simulink model "Citation_FlightGear_v2"  (R2026a)
settings: Solver=ode5  StopTime=40  FixedStep=0.01  EnableMultiTasking=on
InitFcn:
  | run('initcit.m')
  | run('id_init.m')
values from neighbouring files (symbols this model uses):
  cv1 = 20000    [gear_params.m]
  cv2 = cv1    (= 20000)    [gear_params.m]
  cv3 = 4000    [gear_params.m]
  cv4 = 20000    [gear_params.m]
  deltagmax1 = 0.25    [gear_params.m]
  deltagmax2 = deltagmax1    (= 0.25)    [gear_params.m]
  deltagmax3 = 0.24    [gear_params.m]
  deltagmax4 = 0.02    [gear_params.m]
  kt1 = 525020    [gear_params.m]
  kt2 = kt1    (= 525020)    [gear_params.m]
  kt3 = 457050    [gear_params.m]
  murol = 0.03*10    (= 0.3)    [gear_params.m]
  P1 = 2000    [gear_params.m]
  P2 = P1    (= 2000)    [gear_params.m]
  P3 = 2550    [gear_params.m]
  P4 = 40000    [gear_params.m]
  PL0 = 10000*eye(6)    [id_init.m]
  PM0 = 10000*eye(4)    [id_init.m]
  PN0 = 10000*eye(6)    [id_init.m]
  PX0 = 10000*eye(5)    [id_init.m]
  PY0 = 10000*eye(6)    [id_init.m]
  PZ0 = 10000*eye(4)    [id_init.m]
  thetaL0 = zeros(6,1)    [id_init.m]
  thetaM0 = zeros(4,1)    [id_init.m]
  thetaN0 = zeros(6,1)    [id_init.m]
  thetaX0 = zeros(5,1)    [id_init.m]
  thetaY0 = zeros(6,1)    [id_init.m]
  thetaZ0 = zeros(4,1)    [id_init.m]
  TL = 7.0875e-06    [id_init.m]    (also in plot_comparison_step_4.m = T_var(4))
  TM = 3.2564e-06    [id_init.m]    (also in plot_comparison_step_4.m = T_var(5))
  TN = 5.4692e-07    [id_init.m]    (also in plot_comparison_step_4.m = T_var(6))
  TX = 2.2784e-06    [id_init.m]    (also in plot_comparison_step_4.m = T_var(1))
  TY = 8.0633e-07    [id_init.m]    (also in plot_comparison_step_4.m = T_var(2))
  TZ = 2.8004e-05    [id_init.m]    (also in plot_comparison_step_4.m = T_var(3))
  xl1 = xcg-6.858    [gear_params.m]
  xl2 = xcg-6.858    [gear_params.m]
  xl3 = xcg-2.0752    [gear_params.m]
  xl4 = xcg-12.742    [gear_params.m]
  yl1 = 1.918    [gear_params.m]
  yl2 = -1.918    [gear_params.m]
  yl3 = 0    [gear_params.m]
  yl4 = 0    [gear_params.m]
  zl1 = zcg-1.701    [gear_params.m]
  zl2 = zcg-1.701    [gear_params.m]
  zl3 = zcg-1.7488    [gear_params.m]
  zl4 = zcg-2.78    [gear_params.m]
undefined symbols (not defined in the file or in its folder): chord, Deng, ealphag, ealphas, g0, hDME, hGS, lh, massinit, matbuaf, matdaf, matdam, matdbbf, matdeaf, matdgaf, matdqaf, matduaf, matdwaw, matedhr, mateif, matelhr, matemhr, matemv1, matemv2, matemve, matetam, mateuaf, matfaaf, matfaxl, matff, matibaf, matibb, matibmh, matipaf, matipmh, matiraf, matiuaf, matiwaf, matlaf, matlam, matleaf, matleam, matlgaf, matlqaf, matluaf, matmaaf, matmaam, matmaf, matmam, matmbbf, matmeaf, matmeam, matmgaf, matmqaf, matmrbr, matn1d, matn2d, matnbab, matnbaf, matnbmh ... (+53)
libraries: simulink x12, aerolibfltsims x3, aerolibconvert2 x2, aerolibobsolete x1, aerolibanimutils x1
(part 1 of 5)
settings Model: ExtModeTrigMode=oneshot  ExtModeArmWhenConnect=off  Creator=laurensvaneykeren  LastModifiedBy=eltjo
settings DataIOCC: SignalLoggingSaveFormat=ModelDataLogs  SignalLoggingName=sigsOut
settings OptimizationCC: BooleanDataType=off
settings DebuggingCC: SaveWithParameterizedLinksMsg=none  UnderspecifiedInitializationDetection=Classic  SignalResolutionControl=TryResolveAllWithWarning  MultiTaskDSMMsg=warning  MultiTaskCondExecSysMsg=none
settings HardwareCC: ProdHWDeviceType=32-bit Generic  TargetUnknown=on
settings RTWCC: SystemTargetFile=grt_malloc.tlc  GenCodeOnly=on  TemplateMakefile=grt_malloc_default_tmf
settings GRTTargetCC: UseMalloc=on  CombineOutputUpdateFcns=off  GRTInterface=on

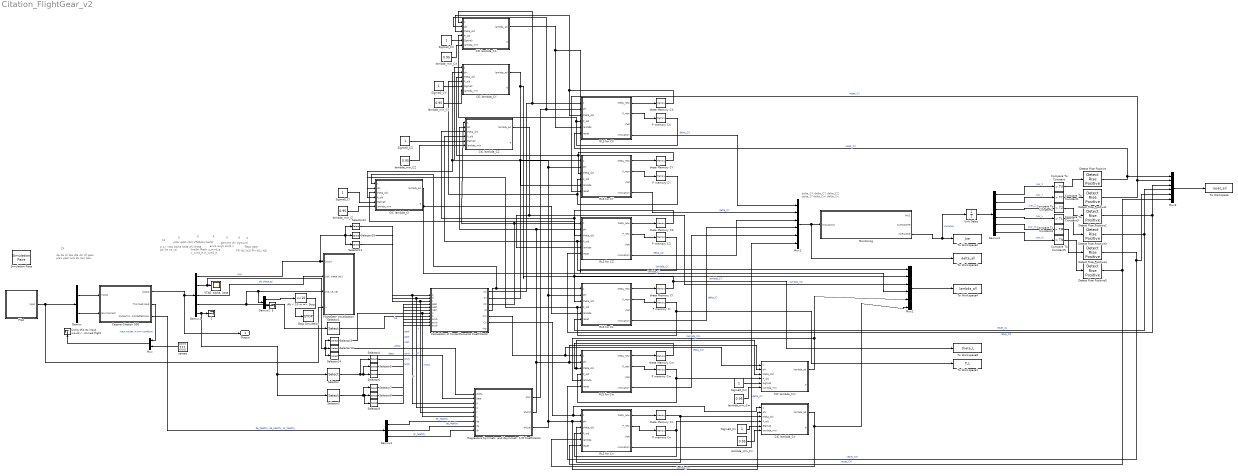
== system Citation_FlightGear_v2 ==
  note: de
      | da
      | dr
      | dte
      | dta
      | dtr
      | df
      | gear
      | pla1
      | pla2
      | turb 8x
      | terr elev
  note: p
      | q
      | r
      | vtas
      | alpha
      | beta
      | phi
      | theta
      | psi
      | he
      | xe
      | ye
  note: pdot
      | qdot
      | rdot
      | VTASdot
      | hedot
  note: hradio
      | Mach
      | u_wind_e
      | v_wind_e
      | w_wind_e
  note: anxb
      | anyb
      | anzb
      | n
  note: gamma
      | chi
      | Vground
  note: flaps
      | gear
  note: FFl
      | N1l
      | N2l
      | FFr
      | N1r
      | N2r
  note: 12
  note: 5
  note: 5
  note: 4
  note: 3
  note: 6
  note: 2
  note: 19
  note: delta_CX
      | delta_CY
      | delta_CZ
      | delta_Cl
      | delta_Cm
      | delta_Cn
  2 : Terminator
  3 : Terminator
  Alt < 10 m => Stop : Fcn  Expr=u<10
  CIC lambda_CX : MATLAB Function  TreatAsAtomicUnit=on
  CIC lambda_CY : MATLAB Function  TreatAsAtomicUnit=on
  CIC lambda_CZ : MATLAB Function  TreatAsAtomicUnit=on
  CIC lambda_Cl : MATLAB Function  TreatAsAtomicUnit=on
  CIC lambda_Cm : MATLAB Function  TreatAsAtomicUnit=on
  CIC lambda_Cn : MATLAB Function  TreatAsAtomicUnit=on
  Calculation of Force/Moments Coefficients : MATLAB Function  TreatAsAtomicUnit=on
  Cessna Citation 500 : Subsystem  mask(Citation Aircraft Model){trimdatafile=}
      mask prompts: trimdatafile "Trim Condition"
      mask init:
      | initcit;
      mask Display:
      | image(imread('Citation.jpg'))
      | port_label('input', 1, 'Inputs')
      | port_label('input', 2, 'Environment')
      | port_label('output', 1, 'Outputs')
      | port_label('output', 2, 'Trim inputs')
  Compare To Constant : simulink/Logic and Bit Operations/Compare To Constant  relop=>  const=TX  OutDataTypeStr=boolean
  Compare To Constant1 : simulink/Logic and Bit Operations/Compare To Constant  relop=>  const=TY  OutDataTypeStr=boolean
  Compare To Constant2 : simulink/Logic and Bit Operations/Compare To Constant  relop=>  const=TZ  OutDataTypeStr=boolean
  Compare To Constant3 : simulink/Logic and Bit Operations/Compare To Constant  relop=>  const=TL  OutDataTypeStr=boolean
  Compare To Constant4 : simulink/Logic and Bit Operations/Compare To Constant  relop=>  const=TM  OutDataTypeStr=boolean
  Compare To Constant5 : simulink/Logic and Bit Operations/Compare To Constant  relop=>  const=TN  OutDataTypeStr=boolean
  Demux : Demux  Outputs=[10 9]
      settings: DisplayOption=none
  Demux1 : Demux  Outputs=[3 3 3 3 25]
      settings: DisplayOption=none
  Demux2 : Demux  Outputs=[1 2]
  Demux3 : Demux  Outputs=3
  Demux4 : Demux  Outputs=6
  Detect Rise Positive{,1..5} (6 alike) : simulink/Logic and Bit Operations/Detect Rise Positive  vinit=0  OutDataTypeStr=boolean
  FlightGear Visualisation : Subsystem
  Monitoring : Subsystem
  Mux : Mux  Inputs=2
  Mux1 : Mux  Inputs=6
  Mux2 : Mux  Inputs=6
  Mux3 : Mux  Inputs=6
  P memory CX : Memory  InitialCondition=PX0
  P memory CY : Memory  InitialCondition=PY0
  P memory CZ : Memory  InitialCondition=PZ0
  P memory Cl : Memory  InitialCondition=PL0
  P memory Cm : Memory  InitialCondition=PM0
  P memory Cn : Memory  InitialCondition=PN0
  Pilot : Subsystem
  RLS for CL : MATLAB Function  TreatAsAtomicUnit=on
  RLS for CX : MATLAB Function  TreatAsAtomicUnit=on
  RLS for CY : MATLAB Function  TreatAsAtomicUnit=on
  RLS for CZ : MATLAB Function  TreatAsAtomicUnit=on
  RLS for Cm : MATLAB Function  TreatAsAtomicUnit=on
  RLS for Cn : MATLAB Function  TreatAsAtomicUnit=on
  Regressors Symmetr. and Asymmetr. F/M Coefficients : MATLAB Function  TreatAsAtomicUnit=on
  Selector : Selector  InputPortWidth=25  IndexOptions=Index vector (dialog)  Indices=[1 2 3]  OutputSizes=1
  Selector1 : Selector  InputPortWidth=3  IndexOptions=Index vector (dialog)  Indices=1  OutputSizes=1
  Selector{5,8,10,13} (4 alike) : Selector  InputPortWidth=3  IndexOptions=Index vector (dialog)  Indices=[2]  OutputSizes=1
  Selector{6,9,11,14} (4 alike) : Selector  InputPortWidth=3  IndexOptions=Index vector (dialog)  Indices=[3]  OutputSizes=1
  Selector{3..4,7,12} (4 alike) : Selector  InputPortWidth=3  IndexOptions=Index vector (dialog)  Indices=[1]  OutputSizes=1
  Selector2 : Selector  InputPortWidth=25  IndexOptions=Index vector (dialog)  Indices=[11 12 13]  OutputSizes=1
  Sigma0_CX : Constant
  Sigma0_CY : Constant
  Sigma0_CZ : Constant
  Sigma0_Cl : Constant
  Sigma0_Cm : Constant
  Sigma0_Cn : Constant
  Simulation Pace : aerolibanimutils/Simulation Pace  SimulationPace=1  SleepMode=MATLAB Thread  OutputPaceError=off  SampleTime=-1
      settings: AttributesFormatString=%<SimulationPace> sec/sec
  Stop Simulation : Stop
  To Workspace : ToWorkspace  VariableName=reset_all  SaveFormat=Timeseries  SampleTime=-1
  To Workspace1 : ToWorkspace  VariableName=P_L  SaveFormat=Timeseries  SampleTime=-1
  To Workspace2 : ToWorkspace  VariableName=Jvar  SaveFormat=Timeseries  SampleTime=-1
  To Workspace3 : ToWorkspace  VariableName=delta_all  SaveFormat=Timeseries  SampleTime=-1
  To Workspace4 : ToWorkspace  VariableName=lambda_all  SaveFormat=Timeseries  SampleTime=-1
  To Workspace8 : ToWorkspace  VariableName=theta_L  SaveFormat=Timeseries  SampleTime=-1
  Unit Delay : UnitDelay  SampleTime=0.01
  Using this as input would result in trimmed flight : Terminator
  "VTAS, alpha, beta" : Scope
      settings: ActiveDisplayYMinimum=-192.0765592563377  ActiveDisplayYMaximum=190.51852643229006  DataLoggingVariableName=ScopeData7
  lambda_min_CX : Constant  Value=0.95
  lambda_min_CY : Constant  Value=0.95
  lambda_min_CZ : Constant  Value=0.95
  lambda_min_Cl : Constant  Value=0.95
  lambda_min_Cm : Constant  Value=0.95
  lambda_min_Cn : Constant  Value=0.95
  theta Memory CX : Memory  InitialCondition=thetaX0
  theta Memory CY : Memory  InitialCondition=thetaY0
  theta Memory CZ : Memory  InitialCondition=thetaZ0
  theta Memory Cl : Memory  InitialCondition=thetaL0
  theta Memory Cm : Memory  InitialCondition=thetaM0
  theta Memory Cn : Memory  InitialCondition=thetaN0
  zeroes : Constant  Value=[0 0 0 0 0 0 0 0 0]
  Output : Outport
  wires:
  Demux/1 -> Cessna Citation 500/1(Inputs)
  Cessna Citation 500/1(output) -> Demux1/1, Output/1
  Demux/2 -> Cessna Citation 500/2(Environment)
  Cessna Citation 500/2(Trimmed input) -> Mux/1  "Input values in trim condition"
  zeroes/1 -> Mux/2
  Mux/1 -> Using this as input would result in trimmed flight/1
  Demux1/1 -> Selector11/1, Selector12/1, Selector10/1, FlightGear Visualisation/1("[p,q,r]")  "p,q,r"
  Demux1/2 -> Selector14/1, Selector3/1, Selector13/1, "VTAS, alpha, beta"/1
  Alt < 10 m => Stop/1 -> Stop Simulation/1
  Demux1/5 -> Selector2/1, Selector/1, 2/1
  Demux1/4 -> Selector1/1, Demux2/1, FlightGear Visualisation/3("[he, xe, ye]")
  Demux2/1 -> Alt < 10 m => Stop/1
  Pilot/1(Input) -> FlightGear Visualisation/4(u), Demux/1
  Demux2/2 -> 3/1
  Demux1/3 -> FlightGear Visualisation/2(" [phi, theta, psi]")  "phi,theta,psi"
  Cessna Citation 500/3(Outport SysID Deflections) -> Demux3/1  "de_healthy, da_healthy, dr_healthy"
  Selector1/1 -> Calculation of Force/Moments Coefficients/8(h)  "he"
  Selector3/1 -> Regressors Symmetr. and Asymmetr. F/M Coefficients/6(V), Calculation of Force/Moments Coefficients/7(V)  "VTAS"
  Selector/1 -> Selector4/1, Selector5/1, Selector6/1
  Selector4/1 -> Calculation of Force/Moments Coefficients/4(pdot)  "pdot"
  Selector5/1 -> Calculation of Force/Moments Coefficients/5(qdot)  "qdot"
  Selector6/1 -> Calculation of Force/Moments Coefficients/6(rdot)  "rdot"
  Selector7/1 -> Calculation of Force/Moments Coefficients/9(anxb)  "anxb"
  Selector9/1 -> Calculation of Force/Moments Coefficients/11(anzb)  "anzb"
  Selector8/1 -> Calculation of Force/Moments Coefficients/10(anyb)  "anyb"
  Selector2/1 -> Selector9/1, Selector8/1, Selector7/1
  Selector12/1 -> Regressors Symmetr. and Asymmetr. F/M Coefficients/3(p), Calculation of Force/Moments Coefficients/1(p)  "p"
  Selector10/1 -> Regressors Symmetr. and Asymmetr. F/M Coefficients/4(q), Calculation of Force/Moments Coefficients/2(q)  "q"
  Selector11/1 -> Regressors Symmetr. and Asymmetr. F/M Coefficients/5(r), Calculation of Force/Moments Coefficients/3(r)  "r"
  Selector13/1 -> Regressors Symmetr. and Asymmetr. F/M Coefficients/1(alpha)  "alpha"
  Selector14/1 -> Regressors Symmetr. and Asymmetr. F/M Coefficients/2(beta)  "beta"
  Demux3/1 -> Regressors Symmetr. and Asymmetr. F/M Coefficients/7(de)  "de_healthy"
  Demux3/2 -> Regressors Symmetr. and Asymmetr. F/M Coefficients/8(da)  "da_healthy"
  Demux3/3 -> Regressors Symmetr. and Asymmetr. F/M Coefficients/9(dr)  "dr_healthy"
  Regressors Symmetr. and Asymmetr. F/M Coefficients/3(phiLat) -> CIC lambda_Cn/2(phi), RLS for Cn/2(phi), RLS for CL/2(phi), RLS for CY/2(phi), CIC lambda_Cl/2(phi), CIC lambda_CY/2(phi)
  RLS for Cn/1(theta_new) -> theta Memory Cn/1
  theta Memory Cn/1 -> RLS for Cn/3(theta_old), CIC lambda_Cn/3(theta_old)
  RLS for Cn/2(P_new) -> P memory Cn/1
  P memory Cn/1 -> RLS for Cn/4(P_old), CIC lambda_Cn/4(P_old)
  Calculation of Force/Moments Coefficients/1(CX) -> CIC lambda_CX/1(z), RLS for CX/1(z)
  P memory CX/1 -> CIC lambda_CX/4(P_old), RLS for CX/4(P_old)
  theta Memory CX/1 -> CIC lambda_CX/3(theta_old), RLS for CX/3(theta_old)
  RLS for CX/2(P_new) -> P memory CX/1
  RLS for CX/1(theta_new) -> theta Memory CX/1
  Regressors Symmetr. and Asymmetr. F/M Coefficients/1(phiX) -> CIC lambda_CX/2(phi), RLS for CX/2(phi)
  P memory CY/1 -> CIC lambda_CY/4(P_old), RLS for CY/4(P_old)
  theta Memory CY/1 -> CIC lambda_CY/3(theta_old), RLS for CY/3(theta_old)
  RLS for CY/2(P_new) -> P memory CY/1
  RLS for CY/1(theta_new) -> theta Memory CY/1
  Calculation of Force/Moments Coefficients/2(CY) -> RLS for CY/1(z), CIC lambda_CY/1(z)
  P memory CZ/1 -> RLS for CZ/4(P_old), CIC lambda_CZ/4(P_old)
  theta Memory CZ/1 -> CIC lambda_CZ/3(theta_old), RLS for CZ/3(theta_old)
  CIC lambda_CZ/1(lambda_ad) -> RLS for CZ/5(lambda), Mux2/3  "lambda_CZ"
  RLS for CZ/2(P_new) -> P memory CZ/1
  RLS for CZ/1(theta_new) -> theta Memory CZ/1
  Calculation of Force/Moments Coefficients/3(CZ) -> RLS for CZ/1(z), CIC lambda_CZ/1(z)
  Regressors Symmetr. and Asymmetr. F/M Coefficients/2(phiZM) -> CIC lambda_Cm/2(phi), RLS for Cm/2(phi), RLS for CZ/2(phi), CIC lambda_CZ/2(phi)
  P memory Cl/1 -> To Workspace1/1, CIC lambda_Cl/4(P_old), RLS for CL/4(P_old)
  theta Memory Cl/1 -> To Workspace8/1, RLS for CL/3(theta_old), CIC lambda_Cl/3(theta_old)
  CIC lambda_Cl/1(lambda_ad) -> Mux2/4, RLS for CL/5(lambda)  "lambda_Cl"
  RLS for CL/2(P_new) -> P memory Cl/1
  RLS for CL/1(theta_new) -> theta Memory Cl/1
  P memory Cm/1 -> RLS for Cm/4(P_old), CIC lambda_Cm/4(P_old)
  theta Memory Cm/1 -> CIC lambda_Cm/3(theta_old), RLS for Cm/3(theta_old)
  RLS for Cm/2(P_new) -> P memory Cm/1
  RLS for Cm/1(theta_new) -> theta Memory Cm/1
  Calculation of Force/Moments Coefficients/4(Cl) -> CIC lambda_Cl/1(z), RLS for CL/1(z)
  Calculation of Force/Moments Coefficients/5(Cm) -> CIC lambda_Cm/1(z), RLS for Cm/1(z)
  Calculation of Force/Moments Coefficients/6(Cn) -> CIC lambda_Cn/1(z), RLS for Cn/1(z)
  RLS for CX/4(innovation) -> Mux1/1  "delta_CX"
  RLS for CY/4(innovation) -> Mux1/2  "delta_CY"
  RLS for CZ/4(innovation) -> Mux1/3  "delta_CZ"
  RLS for CL/4(innovation) -> Mux1/4  "delta_Cl"
  RLS for Cm/4(innovation) -> Mux1/5  "delta_Cm"
  RLS for Cn/4(innovation) -> Mux1/6  "delta_Cn"
  Mux1/1 -> To Workspace3/1, Monitoring/1(innovations)
  Sigma0_CX/1 -> CIC lambda_CX/5(Sigma0)
  lambda_min_CX/1 -> CIC lambda_CX/6(lambda_min)
  CIC lambda_CX/1(lambda_ad) -> Mux2/1, RLS for CX/5(lambda)  "lambda_CX"
  Sigma0_CY/1 -> CIC lambda_CY/5(Sigma0)
  lambda_min_CY/1 -> CIC lambda_CY/6(lambda_min)
  CIC lambda_CY/1(lambda_ad) -> Mux2/2, RLS for CY/5(lambda)  "lambda_CY"
  Sigma0_CZ/1 -> CIC lambda_CZ/5(Sigma0)
  lambda_min_CZ/1 -> CIC lambda_CZ/6(lambda_min)
  Sigma0_Cl/1 -> CIC lambda_Cl/5(Sigma0)
  lambda_min_Cl/1 -> CIC lambda_Cl/6(lambda_min)
  Sigma0_Cm/1 -> CIC lambda_Cm/5(Sigma0)
  lambda_min_Cm/1 -> CIC lambda_Cm/6(lambda_min)
  CIC lambda_Cm/1(lambda_ad) -> Mux2/5, RLS for Cm/5(lambda)  "lambda_Cm"
  Sigma0_Cn/1 -> CIC lambda_Cn/5(Sigma0)
  lambda_min_Cn/1 -> CIC lambda_Cn/6(lambda_min)
  CIC lambda_Cn/1(lambda_ad) -> Mux2/6, RLS for Cn/5(lambda)  "lambda_Cn"
  Monitoring/3(VARIANCE) -> Unit Delay/1, To Workspace2/1  "Variance"
  Mux2/1 -> To Workspace4/1
  Demux4/1 -> Compare To Constant/1  "Jvar_X"
  Demux4/2 -> Compare To Constant1/1  "Jvar_Y"
  Demux4/3 -> Compare To Constant2/1  "Jvar_Z"
  Demux4/4 -> Compare To Constant3/1  "Jvar_L"
  Demux4/5 -> Compare To Constant4/1  "Jvar_M"
  Demux4/6 -> Compare To Constant5/1  "Jvar_N"
  Compare To Constant/1 -> Detect Rise Positive/1
  Compare To Constant1/1 -> Detect Rise Positive1/1
  Compare To Constant2/1 -> Detect Rise Positive2/1
  Compare To Constant3/1 -> Detect Rise Positive3/1
  Compare To Constant5/1 -> Detect Rise Positive5/1
  Compare To Constant4/1 -> Detect Rise Positive4/1
  Detect Rise Positive/1 -> RLS for CX/6(reset), Mux3/1  "reset_CX"
  Detect Rise Positive1/1 -> Mux3/2, RLS for CY/6(reset)  "reset_CY"
  Detect Rise Positive2/1 -> RLS for CZ/6(reset), Mux3/3  "reset_CZ"
  Detect Rise Positive3/1 -> RLS for CL/6(reset), Mux3/4  "reset_CL"
  Detect Rise Positive4/1 -> Mux3/5, RLS for Cm/6(reset)  "reset_CM"
  Detect Rise Positive5/1 -> RLS for Cn/6(reset), Mux3/6  "reset_CN"
  Mux3/1 -> To Workspace/1
  Unit Delay/1 -> Demux4/1

== system Citation_FlightGear_v2/Cessna Citation 500 ==
  note: p
      | q
      | r
      | vtas
      | alpha
      | beta
      | phi
      | theta
      | psi
      | he
      | xe
      | ye
  note: de
      | da
      | dr
      | dte
      | dta
      | dtr
      | df
      | gear
      | pla1
      | pla2
  note: pdot
      | qdot
      | rdot
      | VTASdot
      | hedot
  note: hradio
      | Mach
      | u_wind_e
      | v_wind_e
      | w_wind_e
  note: anxb
      | anyb
      | anzb
      | n
  note: gamma
      | chi
      | Vground
  note: turb 8x
      | terr_elev
  note: flaps
      | gear
  note: de
      | da
      | dr
      | dte
      | dta
      | dtr
      | df
      | gear
      | pla1
      | pla2
  note: FFl
      | N1l
      | N2l
      | FFr
      | N1r
      | N2r
  Inputs : Inport
  Environment : Inport  Port=2
  Actuators : Subsystem
  Citation model DASMAT : Subsystem
  Controllers : Subsystem
  Demux4 : Demux  Outputs=[8 2]
      settings: DisplayOption=none
  Mux1 : Mux  Inputs=7
  Mux2 : Mux  Inputs=2
  trim conditions : Subsystem
  ua sel : Selector  IndexOptions=Index vector (dialog)  Indices=[5 6]  OutputSizes=1
  xdot sel : Selector  IndexOptions=Index vector (dialog)  Indices=[1 2 3 4 10]  OutputSizes=1
  yacc sel : Selector  IndexOptions=Index vector (dialog)  Indices=[4 5 6 15]  OutputSizes=1
  yair sel : Selector  IndexOptions=Index vector (dialog)  Indices=[6 9 22 23 24]  OutputSizes=1
  yfp sel : Selector  IndexOptions=Index vector (dialog)  Indices=[1 2 15]  OutputSizes=1
  ypp sel : Selector  IndexOptions=Index vector (dialog)  Indices=[2 3 4 13 14 15]  OutputSizes=1
  output : Outport
  Trimmed input : Outport  Port=2
  Outport SysID Deflections : Outport  Port=3
  wires:
  Mux1/1 -> output/1
  Citation model DASMAT/1(x) -> Mux1/1, Controllers/1(state)
  Inputs/1 -> Controllers/2(inputs)
  Demux4/1 -> Citation model DASMAT/1(ua), ua sel/1
  Demux4/2 -> Citation model DASMAT/2(ut)
  Environment/1 -> Citation model DASMAT/3(Environment)
  Citation model DASMAT/3(yair) -> yair sel/1
  yair sel/1 -> Mux1/3
  Citation model DASMAT/2(xdot) -> xdot sel/1
  xdot sel/1 -> Mux1/2
  yacc sel/1 -> Mux1/4
  Citation model DASMAT/4(yacc) -> yacc sel/1
  yfp sel/1 -> Mux1/5
  Citation model DASMAT/5(yfp) -> yfp sel/1
  Actuators/1(Out) -> Demux4/1
  trim conditions/1(ua) -> Mux2/1
  trim conditions/2(ut) -> Mux2/2
  Mux2/1 -> Trimmed input/1
  Controllers/1(control inputs) -> Actuators/1(In)
  ua sel/1 -> Mux1/7
  Citation model DASMAT/6(ypp) -> ypp sel/1
  ypp sel/1 -> Mux1/6
  Actuators/2(Outport SysID Deflections) -> Outport SysID Deflections/1

== system Citation_FlightGear_v2/FlightGear Visualisation ==
  "[p,q,r]" : Inport
  " [phi, theta, psi]" : Inport  Port=2
  "[he, xe, ye]" : Inport  Port=3
  u : Inport  Port=4
  Constant : Constant  Value=0
  Generate Run Script : aerolibfltsims/Generate Run Script  Architecture=Win64  dataFlow=Send  GeometryModelName=Yak-36  AirportId=KSFO  RunwayId=10L  InitialAltitude=7224  InitialHeading=113  OffsetDistance=4.72  OffsetAzimuth=0  InstallScenery=off  DisableShaders=off  OriginAddress=127.0.0.1  DestinationPort=5502  OriginPort=5505  LocalAddress=127.0.0.1  OutputFileName=runfg30.bat  FlightGearBaseDirectory=D:\Program Files\FlightGear3.0
  "P, Q, R" : Scope
      settings: ActiveDisplayYMinimum=-2.789820175659862  ActiveDisplayYMaximum=3.3807681055005783  DataLoggingVariableName=ScopeData2
  Send net_fdm Packet to FlightGear : aerolibfltsims/Send net_fdm Packet to FlightGear  DestinationIpAddress=127.0.0.1  DestinationPort=5502  LocalIpPort=-1  varLen=off  SampleTime=-1
  Subsystem : Subsystem
  Sum1 : Sum  Inputs=|++
  "h, posN,posE " : Scope
      settings: TimeSpan=10  ActiveDisplayYMinimum=-20000  ActiveDisplayYMaximum=10000  DataLoggingVariableName=ScopeData5
  "h, posN,posE, offsets" : Constant  Value=[0 -1000 2000]
  phi,theta,psi : Scope
      settings: ActiveDisplayYMinimum=-14.69567  ActiveDisplayYMaximum=1.72975  DataLoggingVariableName=ScopeData3
  wires:
  "h, posN,posE, offsets"/1 -> Sum1/2
  Sum1/1 -> "h, posN,posE "/1, Subsystem/3(Xe)
  Constant/1 -> Subsystem/4(href)
  u/1 -> Subsystem/5(u)
  Subsystem/1(FG Packet) -> Send net_fdm Packet to FlightGear/1
  "[he, xe, ye]"/1 -> Sum1/1
  "[p,q,r]"/1 -> "P, Q, R"/1, Subsystem/1(pqr)
  " [phi, theta, psi]"/1 -> phi,theta,psi/1, Subsystem/2(phi theta psi)

== system Citation_FlightGear_v2/Monitoring ==
  note: MA2 = moving average of the squared innovation
      | AUTOCORR = autocorrelation function
      | VARIANCE = spectral analysis
  innovations : Inport
  Monitoring Metrics : MATLAB Function  TreatAsAtomicUnit=on
  Zero-Order Hold : ZeroOrderHold  SampleTime=0.01
  MA2 : Outport
  AUTOCORR : Outport  Port=2
  VARIANCE : Outport  Port=3
  wires:
  innovations/1 -> Zero-Order Hold/1
  Zero-Order Hold/1 -> Monitoring Metrics/1(innovations)
  Monitoring Metrics/1(MA2) -> MA2/1
  Monitoring Metrics/2(AUTOCORR) -> AUTOCORR/1
  Monitoring Metrics/3(VARIANCE) -> VARIANCE/1

== system Citation_FlightGear_v2/Pilot ==
  note: de
      | da
      | dr
      | dte
      | dta
      | dtr
      | df
      | gear
      | pla1
      | pla2
      | turb 8x
      | terr elev
  Virtual Joystick (if you don't have a real one!) : Subsystem
  Input : Outport
  wires:
  Virtual Joystick (if you don't have a real one!)/1(Virtual joystick input) -> Input/1

== system Citation_FlightGear_v2/Cessna Citation 500/Actuators ==
  note: de
      | da
      | dr
      | dte
      | dta
      | dtr
      | df
      | gear
      | pla1
      | pla2
  note: de
      | da
      | dr
      | dte
      | dta
      | dtr
      | df
      | gear
      | pla1
      | pla2
  In : Inport
  Add : Sum
  Constant : Constant  Value=-0.28
  Demux : Demux  Outputs=10
      settings: DisplayOption=none
  Failure Activation : Step  Time=100  SampleTime=0
  Gain : Gain  Gain=0.5
  Mux : Mux  Inputs=10
  Mux1 : Mux  Inputs=3
  Switch : Switch  Criteria=u2 > Threshold  Threshold=0.5  SaturateOnIntegerOverflow=off  InputSameDT=off
  To Workspace : ToWorkspace  VariableName=failure_activation  SaveFormat=Timeseries  SampleTime=-1
      settings: Save2DSignal=2-D array (concatenate along first dimension)
  da : Subsystem
  da limits : Saturate  UpperLimit=0.65  LowerLimit=-0.65
  de : Subsystem
  de limits : Saturate  UpperLimit=0.26  LowerLimit=-0.35
  dr : Subsystem
  dr limits : Saturate  UpperLimit=0.38  LowerLimit=-0.38
  flaps : Subsystem
  gear : Subsystem
  Out : Outport
  Outport SysID Deflections : Outport  Port=2
  wires:
  In/1 -> Demux/1
  Mux/1 -> Out/1
  Demux/1 -> de/1(In)
  Demux/2 -> da/1(In)
  Demux/3 -> dr/1(In)
  de/1(Out) -> de limits/1
  da/1(Out) -> da limits/1
  da limits/1 -> Mux1/2, Gain/1, Switch/3  "da_healthy"
  dr/1(Out) -> dr limits/1
  dr limits/1 -> Mux1/3, Mux/3  "dr_healthy"
  de limits/1 -> Mux1/1, Mux/1  "de_healthy"
  Demux/8 -> gear/1(In)
  Demux/7 -> flaps/1(In)
  Demux/9 -> Mux/9
  Demux/10 -> Mux/10
  flaps/1(Out) -> Mux/7
  gear/1(Out) -> Mux/8
  Demux/4 -> Mux/4
  Demux/5 -> Mux/5
  Demux/6 -> Mux/6
  Gain/1 -> Add/2
  Constant/1 -> Add/1
  Add/1 -> Switch/1  "da_failed"
  Switch/1 -> Mux/2  "da_actual"
  Failure Activation/1 -> Switch/2, To Workspace/1
  Mux1/1 -> Outport SysID Deflections/1

== system Citation_FlightGear_v2/Cessna Citation 500/Citation model DASMAT ==
  ua : Inport
  ut : Inport  Port=2
  Environment : Inport  Port=3
  AIRCRAFT MODEL : Subsystem
  Mux1 : Mux  Inputs=[8 2 8 12 8]
  Terminator_{16..19} (4 alike) : Terminator
  massinit : Constant  Value=massinit
  x : Outport
  xdot : Outport  Port=2
  yair : Outport  Port=3
  yacc : Outport  Port=4
  yfp : Outport  Port=5
  ypp : Outport  Port=6
  wires:
  AIRCRAFT MODEL/13(FMt) -> Terminator_19/1
  Mux1/1 -> yair/1
  AIRCRAFT MODEL/12(FMag) -> Terminator_17/1
  AIRCRAFT MODEL/11(FMa) -> Terminator_18/1
  AIRCRAFT MODEL/7(gust) -> Mux1/5
  AIRCRAFT MODEL/6(wind) -> Mux1/4
  AIRCRAFT MODEL/5(yad2) -> Mux1/3
  AIRCRAFT MODEL/4(yad1) -> Mux1/2
  AIRCRAFT MODEL/3(yatm) -> Mux1/1
  AIRCRAFT MODEL/2(xdot) -> xdot/1
  AIRCRAFT MODEL/1(x) -> x/1
  AIRCRAFT MODEL/10(ys) -> Terminator_16/1
  AIRCRAFT MODEL/9(yfp) -> yfp/1
  AIRCRAFT MODEL/8(yacc) -> yacc/1
  ut/1 -> AIRCRAFT MODEL/2(ut)
  ua/1 -> AIRCRAFT MODEL/1(ua)
  Environment/1 -> AIRCRAFT MODEL/4(Environment)
  AIRCRAFT MODEL/14(ypp) -> ypp/1
  massinit/1 -> AIRCRAFT MODEL/3(massinit)

== system Citation_FlightGear_v2/Cessna Citation 500/Controllers ==
  state : Inport
  inputs : Inport  Port=2
  A/T disabled : Gain  Gain=0  SaturateOnIntegerOverflow=on  OutDataTypeStr=Inherit: Same as input  ParamDataTypeStr=Inherit: Same as input
  Yaw damper : Subsystem
  add controller outputs to pilot inputs : Sum  Inputs=|+|+|+|  SaturateOnIntegerOverflow=on
  auto throttle : Subsystem
  control inputs : Outport
  wires:
  state/1 -> Yaw damper/1(state), auto throttle/1(state)
  inputs/1 -> Yaw damper/2(inputs), add controller outputs to pilot inputs/3, auto throttle/2(inputs)
  add controller outputs to pilot inputs/1 -> control inputs/1
  Yaw damper/1(controller output) -> add controller outputs to pilot inputs/1
  auto throttle/1(controller output) -> A/T disabled/1
  A/T disabled/1 -> add controller outputs to pilot inputs/2

== system Citation_FlightGear_v2/Cessna Citation 500/trim conditions ==
  PLA1/Tx1 : Constant  Value=ut0(1)
  PLA2/Tx2 : Constant  Value=ut0(2)
  control inputs : Mux  Inputs=8
      settings: DisplayOption=signals
  deltaa : Constant  Value=u0(2)
  deltae : Constant  Value=u0(1)
  deltaf : Constant  Value=u0(7)
  deltar : Constant  Value=u0(3)
  deltata : Constant  Value=u0(5)
  deltate : Constant  Value=u0(4)
  deltatr : Constant  Value=u0(6)
  engine inputs : Mux  Inputs=2
      settings: DisplayOption=signals
  lgsw : Constant  Value=u0(8)
  ua : Outport
  ut : Outport  Port=2
  wires:
  deltaf/1 -> control inputs/7  "df"
  engine inputs/1 -> ut/1
  deltatr/1 -> control inputs/6  "dtr"
  deltata/1 -> control inputs/5  "dta"
  control inputs/1 -> ua/1
  PLA1/Tx1/1 -> engine inputs/1  "pla1"
  PLA2/Tx2/1 -> engine inputs/2  "pla2"
  deltae/1 -> control inputs/1  "de"
  deltaa/1 -> control inputs/2  "da"
  deltar/1 -> control inputs/3  "dr"
  deltate/1 -> control inputs/4  "dte"
  lgsw/1 -> control inputs/8  "lg"

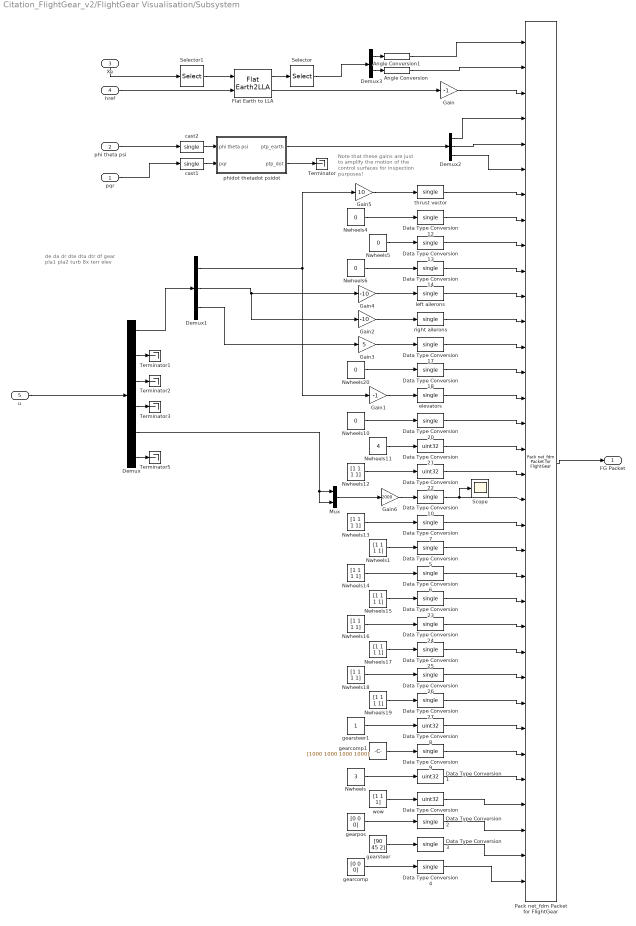
== system Citation_FlightGear_v2/FlightGear Visualisation/Subsystem ==
  note: Note that these gains are just to amplify the motion of the control surfaces for inspection purposes!
  note: de
      | da
      | dr
      | dte
      | dta
      | dtr
      | df
      | gear
      | pla1
      | pla2
      | turb 8x
      | terr elev
  pqr : Inport
  phi theta psi : Inport  Port=2
  Xe : Inport  Port=3
  href : Inport  Port=4
  u : Inport  Port=5
  Angle Conversion : aerolibconvert2/Angle Conversion  IU=deg  OU=rad
  Angle Conversion1 : aerolibconvert2/Angle Conversion  IU=deg  OU=rad
  Data Type Conversion{,1,8,21..22} (5 alike) : DataTypeConversion  OutDataTypeStr=uint32  SaturateOnIntegerOverflow=off  RndMeth=Floor
  Data Type Conversion{2..7,9..10,12..14,17..18,20,23..27} (19 alike) : DataTypeConversion  OutDataTypeStr=single  SaturateOnIntegerOverflow=off  RndMeth=Floor
  Demux : Demux  Outputs=[3 3 1 1 2 9]
  Demux1 : Demux  Outputs=[1 1 1]
  Demux2 : Demux  Outputs=3
  Demux3 : Demux  Outputs=2
  Flat Earth to LLA : FlatEarth2LLA  R=6378137  LL0=[37.7889 -122.4778]
  Gain : Gain  Gain=-1
  Gain1 : Gain  Gain=-1
  Gain2 : Gain  Gain=-10
  Gain3 : Gain  Gain=5
  Gain4 : Gain  Gain=-10
  Gain5 : Gain  Gain=10
  Gain6 : Gain  Gain=2000
  Mux : Mux  Inputs=2
  Nwheels : Constant  Value=3
  Nwheels{1,12..19} (9 alike) : Constant  Value=[1 1 1 1]
  Nwheels{4..6,10,20} (5 alike) : Constant  Value=0
  Nwheels11 : Constant  Value=4
  Pack net_fdm Packet for FlightGear : aerolibfltsims/Pack net_fdm Packet for FlightGear  FlightGearVersion=v2016.1  ShowPositionAttitudeInputs=on  ShowVelocityAccelerationInputs=off  ShowControlSurfacePositionInputs=on  ShowEngineFuelInputs=on  ShowLandingGearInputs=on  ShowEnvironmentInputs=off  SampleTime=-1  packetVersion=24
  Scope : Scope
      settings: ActiveDisplayYMinimum=-1.2099758283130364E+6  ActiveDisplayYMaximum=2.11709328029719E+6
  Selector : Selector  InputPortWidth=2  IndexOptions=Index vector (dialog)  Indices=[2 1]  OutputSizes=1
  Selector1 : Selector  InputPortWidth=3  IndexOptions=Index vector (dialog)  Indices=[2 3 1]  OutputSizes=1
  Terminator{,1..3,5} (5 alike) : Terminator
  cast1 : DataTypeConversion  OutDataTypeStr=single  RndMeth=Floor
  cast2 : DataTypeConversion  OutDataTypeStr=single  RndMeth=Floor
  elevators : DataTypeConversion  OutDataTypeStr=single  SaturateOnIntegerOverflow=off  RndMeth=Floor
  gearcomp : Constant  Value=[0 0 0]
  gearcomp1 : Constant  Value=[1000 1000 1000 1000]
  gearpos : Constant  Value=[0 0 0]  VectorParams1D=off
  gearsteer : Constant  Value=[90 45 2]
  gearsteer1 : Constant
  left ailerons : DataTypeConversion  OutDataTypeStr=single  SaturateOnIntegerOverflow=off  RndMeth=Floor
  phidot thetadot psidot : Subsystem
  right ailerons : DataTypeConversion  OutDataTypeStr=single  SaturateOnIntegerOverflow=off  RndMeth=Floor
  thrust vector : DataTypeConversion  OutDataTypeStr=single  SaturateOnIntegerOverflow=off  RndMeth=Floor
  wow : Constant  Value=[1 1 1]
  FG Packet : Outport  VectorParamsAs1DForOutWhenUnconnected=off
  wires:
  Pack net_fdm Packet for FlightGear/1 -> FG Packet/1
  href/1 -> Flat Earth to LLA/2
  Flat Earth to LLA/1 -> Selector/1
  Selector/1 -> Demux3/1
  Demux3/1 -> Angle Conversion1/1
  Demux3/2 -> Angle Conversion/1
  Angle Conversion1/1 -> Pack net_fdm Packet for FlightGear/1
  phidot thetadot psidot/1(ptp_earth) -> Demux2/1
  Demux2/1 -> Pack net_fdm Packet for FlightGear/4
  Demux2/2 -> Pack net_fdm Packet for FlightGear/5
  Demux2/3 -> Pack net_fdm Packet for FlightGear/6
  phidot thetadot psidot/2(ptp_dot) -> Terminator/1
  pqr/1 -> cast1/1
  Angle Conversion/1 -> Pack net_fdm Packet for FlightGear/2
  Flat Earth to LLA/2 -> Gain/1
  Gain/1 -> Pack net_fdm Packet for FlightGear/3
  Data Type Conversion17/1 -> Pack net_fdm Packet for FlightGear/13
  Data Type Conversion8/1 -> Pack net_fdm Packet for FlightGear/28
  Nwheels13/1 -> Data Type Conversion7/1
  Data Type Conversion25/1 -> Pack net_fdm Packet for FlightGear/25
  left ailerons/1 -> Pack net_fdm Packet for FlightGear/11
  Nwheels15/1 -> Data Type Conversion23/1
  Nwheels19/1 -> Data Type Conversion27/1
  Data Type Conversion12/1 -> Pack net_fdm Packet for FlightGear/8
  Data Type Conversion9/1 -> Pack net_fdm Packet for FlightGear/29
  Demux1/2 -> Gain2/1, Gain4/1
  Data Type Conversion21/1 -> Pack net_fdm Packet for FlightGear/17
  Data Type Conversion14/1 -> Pack net_fdm Packet for FlightGear/10
  Data Type Conversion6/1 -> Pack net_fdm Packet for FlightGear/22
  thrust vector/1 -> Pack net_fdm Packet for FlightGear/7
  Nwheels6/1 -> Data Type Conversion14/1
  Nwheels12/1 -> Data Type Conversion22/1
  Nwheels14/1 -> Data Type Conversion6/1
  Nwheels5/1 -> Data Type Conversion13/1
  right ailerons/1 -> Pack net_fdm Packet for FlightGear/12
  Data Type Conversion22/1 -> Pack net_fdm Packet for FlightGear/18
  gearcomp1/1 -> Data Type Conversion9/1
  Data Type Conversion13/1 -> Pack net_fdm Packet for FlightGear/9
  Data Type Conversion26/1 -> Pack net_fdm Packet for FlightGear/26
  Nwheels1/1 -> Data Type Conversion5/1
  gearsteer1/1 -> Data Type Conversion8/1
  elevators/1 -> Pack net_fdm Packet for FlightGear/15
  Data Type Conversion18/1 -> Pack net_fdm Packet for FlightGear/14
  Data Type Conversion20/1 -> Pack net_fdm Packet for FlightGear/16
  Nwheels10/1 -> Data Type Conversion20/1
  Xe/1 -> Selector1/1
  Data Type Conversion10/1 -> Scope/1, Pack net_fdm Packet for FlightGear/19
  Nwheels4/1 -> Data Type Conversion12/1
  Data Type Conversion27/1 -> Pack net_fdm Packet for FlightGear/27
  Data Type Conversion4/1 -> Pack net_fdm Packet for FlightGear/34
  gearpos/1 -> Data Type Conversion2/1
  Data Type Conversion2/1 -> Pack net_fdm Packet for FlightGear/32
  Data Type Conversion3/1 -> Pack net_fdm Packet for FlightGear/33
  Nwheels/1 -> Data Type Conversion1/1
  wow/1 -> Data Type Conversion/1
  gearsteer/1 -> Data Type Conversion3/1
  Data Type Conversion1/1 -> Pack net_fdm Packet for FlightGear/30
  gearcomp/1 -> Data Type Conversion4/1
  Data Type Conversion/1 -> Pack net_fdm Packet for FlightGear/31
  Nwheels17/1 -> Data Type Conversion25/1
  Nwheels16/1 -> Data Type Conversion24/1
  Data Type Conversion23/1 -> Pack net_fdm Packet for FlightGear/23
  Data Type Conversion24/1 -> Pack net_fdm Packet for FlightGear/24
  Nwheels11/1 -> Data Type Conversion21/1
  Data Type Conversion7/1 -> Pack net_fdm Packet for FlightGear/20
  Data Type Conversion5/1 -> Pack net_fdm Packet for FlightGear/21
  Nwheels18/1 -> Data Type Conversion26/1
  cast2/1 -> phidot thetadot psidot/1(phi theta psi)
  cast1/1 -> phidot thetadot psidot/2(pqr)
  phi theta psi/1 -> cast2/1
  Demux1/3 -> Gain3/1
  Nwheels20/1 -> Data Type Conversion18/1
  u/1 -> Demux/1
  Gain1/1 -> elevators/1
  Demux1/1 -> Gain1/1, Gain5/1
  Demux/1 -> Demux1/1
  Gain2/1 -> right ailerons/1
  Demux/2 -> Terminator1/1
  Demux/3 -> Terminator2/1
  Demux/4 -> Terminator3/1
  Demux/6 -> Terminator5/1
  Selector1/1 -> Flat Earth to LLA/1
  Gain3/1 -> Data Type Conversion17/1
  Gain4/1 -> left ailerons/1
  Gain5/1 -> thrust vector/1
  Demux/5 -> Mux/1, Mux/2
  Mux/1 -> Gain6/1
  Gain6/1 -> Data Type Conversion10/1

== system Citation_FlightGear_v2/Pilot/Virtual Joystick (if you don't have a real one!) ==
  Mux1 : Mux  Inputs=12
  Virtual Joystick : Subsystem
  da trim1 : Constant  Value=0
  de trim1 : Constant  Value=0
  delta flaps1 : Constant  Value=0
  dr trim1 : Constant  Value=0
  gear (ON=1/OFF=0)1 : Constant  Value=0
  terr elev1 : Constant  Value=0
  turb 8x1 : Constant  Value=zeros(1,8)
  Virtual joystick input : Outport
  wires:
  turb 8x1/1 -> Mux1/11
  da trim1/1 -> Mux1/5
  Virtual Joystick/4(Signal 4) -> Mux1/9, Mux1/10
  Virtual Joystick/1(Signal 1) -> Mux1/1
  dr trim1/1 -> Mux1/6
  Virtual Joystick/3(Signal 3) -> Mux1/3
  Virtual Joystick/2(Signal 2) -> Mux1/2
  gear (ON=1/OFF=0)1/1 -> Mux1/8
  terr elev1/1 -> Mux1/12
  delta flaps1/1 -> Mux1/7
  de trim1/1 -> Mux1/4
  Mux1/1 -> Virtual joystick input/1  "Virtual joystick input"

== system Citation_FlightGear_v2/Cessna Citation 500/Actuators/da ==
  In : Inport
  Gain : Gain  Gain=13  SaturateOnIntegerOverflow=on  OutDataTypeStr=Inherit: Same as input  ParamDataTypeStr=Inherit: Same as input
  Integrator : Integrator  InitialCondition=u0(2)
  Sum : Sum  Inputs=|+-  SaturateOnIntegerOverflow=on
  Out : Outport
  wires:
  Integrator/1 -> Out/1, Sum/2
  In/1 -> Sum/1
  Sum/1 -> Gain/1
  Gain/1 -> Integrator/1

== system Citation_FlightGear_v2/Cessna Citation 500/Actuators/de ==
  In : Inport
  Gain : Gain  Gain=13  SaturateOnIntegerOverflow=on  OutDataTypeStr=Inherit: Same as input  ParamDataTypeStr=Inherit: Same as input
  Integrator : Integrator  InitialCondition=u0(1)
  Sum : Sum  Inputs=|+-  SaturateOnIntegerOverflow=on
  Out : Outport
  wires:
  Integrator/1 -> Out/1, Sum/2
  In/1 -> Sum/1
  Sum/1 -> Gain/1
  Gain/1 -> Integrator/1

== system Citation_FlightGear_v2/Cessna Citation 500/Actuators/dr ==
  In : Inport
  Gain : Gain  Gain=13  SaturateOnIntegerOverflow=on  OutDataTypeStr=Inherit: Same as input  ParamDataTypeStr=Inherit: Same as input
  Integrator : Integrator  InitialCondition=u0(3)
  Sum : Sum  Inputs=|+-  SaturateOnIntegerOverflow=on
  Out : Outport
  wires:
  Integrator/1 -> Out/1, Sum/2
  In/1 -> Sum/1
  Sum/1 -> Gain/1
  Gain/1 -> Integrator/1

== system Citation_FlightGear_v2/Cessna Citation 500/Actuators/flaps ==
  In : Inport
  Gain : Gain  Gain=0.9  SaturateOnIntegerOverflow=on  OutDataTypeStr=Inherit: Same as input  ParamDataTypeStr=Inherit: Same as input
  Integrator : Integrator  InitialCondition=u0(7)
  Sum : Sum  Inputs=|+-  SaturateOnIntegerOverflow=on
  Out : Outport
  wires:
  Integrator/1 -> Out/1, Sum/2
  In/1 -> Sum/1
  Sum/1 -> Gain/1
  Gain/1 -> Integrator/1

== system Citation_FlightGear_v2/Cessna Citation 500/Actuators/gear ==
  In : Inport
  Gain : Gain  Gain=0.6  SaturateOnIntegerOverflow=on  OutDataTypeStr=Inherit: Same as input  ParamDataTypeStr=Inherit: Same as input
  Integrator : Integrator  InitialCondition=u0(8)
  Sum : Sum  Inputs=|+-  SaturateOnIntegerOverflow=on
  Out : Outport
  wires:
  Integrator/1 -> Out/1, Sum/2
  In/1 -> Sum/1
  Sum/1 -> Gain/1
  Gain/1 -> Integrator/1

== system Citation_FlightGear_v2/Cessna Citation 500/Citation model DASMAT/AIRCRAFT MODEL ==
  ua : Inport
  ut : Inport  Port=2
  massinit : Inport  Port=3
  Environment : Inport  Port=4
  AFM : Subsystem
  AIRDATA : Subsystem
  Demux : Demux  Outputs=[8 1]
      settings: DisplayOption=none
  EFM : Subsystem
  EQM : Subsystem
  FM SORT : Subsystem
  GRAVITY : Subsystem
  LANDING GEAR : Subsystem
  OBSERVATIONS : Subsystem
  WIND/TURBULENCE : Subsystem
  x : Outport
  xdot : Outport  Port=2
  yatm : Outport  Port=3
  yad1 : Outport  Port=4
  yad2 : Outport  Port=5
  wind : Outport  Port=6
  gust : Outport  Port=7
  yacc : Outport  Port=8
  yfp : Outport  Port=9
  ys : Outport  Port=10
  FMa : Outport  Port=11
  FMag : Outport  Port=12
  FMt : Outport  Port=13
  ypp : Outport  Port=14
  wires:
  AFM/1(FMa) -> FM SORT/1(FMa), EQM/2(FMa)
  OBSERVATIONS/3(ys) -> ys/1
  OBSERVATIONS/2(yfp) -> yfp/1
  EQM/4(FMtot corrected) -> OBSERVATIONS/4(FMtot)
  EQM/3(yuvw) -> OBSERVATIONS/3(yuvw)
  EFM/1(FMt) -> FM SORT/3(FMt), FMt/1
  AFM/4(FMag) -> FM SORT/2(FMag), FMag/1
  ua/1 -> AFM/2(ua), LANDING GEAR/4(ua)
  ut/1 -> EFM/2(ut)
  OBSERVATIONS/1(yacc) -> yacc/1
  FM SORT/1(FMtot) -> EQM/1("FMtot ")
  EQM/5(FMa corrected) -> OBSERVATIONS/5(FMa), FMa/1
  AFM/2(FMadot) -> EQM/3(FMadot)
  AFM/3(FMbdot) -> EQM/4(FMbdot)
  GRAVITY/1(Fgr) -> FM SORT/4("Fgr "), OBSERVATIONS/6(Fgr)
  massinit/1 -> EFM/3(massinit), AFM/3(massinit), GRAVITY/2(massinit), EQM/5(massinit), OBSERVATIONS/7(massinit), LANDING GEAR/3(massinit)
  AIRDATA/3(yad2) -> EFM/6(yad2), AFM/5(yad2), yad2/1
  AIRDATA/2(yad1) -> AFM/4(yad1), EFM/5(yad1), yad1/1
  AIRDATA/1(yatm) -> yatm/1, GRAVITY/3(yatm), OBSERVATIONS/8(yatm), EFM/4(yatm), AFM/7(yatm)
  EQM/1(x) -> GRAVITY/1("x "), LANDING GEAR/1(x), EFM/1(x), AFM/1(x), WIND/TURBULENCE/1("x "), AIRDATA/1(x), x/1, OBSERVATIONS/1(x)
  WIND/TURBULENCE/1(wind) -> EQM/6(wind), wind/1
  EQM/2(xdot) -> xdot/1, OBSERVATIONS/2(xdot), LANDING GEAR/2(xdot)
  Environment/1 -> Demux/1
  Demux/1 -> gust/1, AFM/6(gust)
  Demux/2 -> AIRDATA/2(terrain elevation), LANDING GEAR/5(terr elev)  "terrain elevation"
  LANDING GEAR/1(Fmt) -> FM SORT/5(Fgear)
  EFM/2(ypp) -> ypp/1

== system Citation_FlightGear_v2/Cessna Citation 500/Controllers/Yaw damper ==
  state : Inport
  inputs : Inport  Port=2
  Gain : Gain  SaturateOnIntegerOverflow=on  OutDataTypeStr=Inherit: Same as input  ParamDataTypeStr=Inherit: Same as input
  Washout : TransferFcn  Numerator=[1 0]  Denominator=[1 1/4]
  dr : Gain  Gain=[0 0 1 0 0 0 0 0 0 0]  SaturateOnIntegerOverflow=on  OutDataTypeStr=Inherit: Same as input  ParamDataTypeStr=Inherit: Same as input
  not used : Terminator
  r  sel : Selector  IndexOptions=Index vector (dialog)  Indices=[3]  OutputSizes=1
  controller output : Outport
  wires:
  Washout/1 -> Gain/1
  dr/1 -> controller output/1
  state/1 -> r  sel/1
  r  sel/1 -> Washout/1  "r"
  inputs/1 -> not used/1
  Gain/1 -> dr/1

== system Citation_FlightGear_v2/Cessna Citation 500/Controllers/auto throttle ==
  state : Inport
  inputs : Inport  Port=2
  Gain : Gain  Gain=0.5  SaturateOnIntegerOverflow=on  OutDataTypeStr=Inherit: Same as input  ParamDataTypeStr=Inherit: Same as input
  Saturation : Saturate  UpperLimit=1.0  LowerLimit=0.0
  Sum : Sum  Inputs=+-|  SaturateOnIntegerOverflow=on
  VTAS ref (trim value) : Constant  Value=x0(4)
  VTAS sel : Selector  IndexOptions=Index vector (dialog)  Indices=[4]  OutputSizes=1
  controller output is later added to pilot input! : Sum  Inputs=|+-  SaturateOnIntegerOverflow=on
  pla1&2 : Gain  Gain=[0 0 0 0 0 0 0 0 1 1]  SaturateOnIntegerOverflow=on  OutDataTypeStr=Inherit: Same as input  ParamDataTypeStr=Inherit: Same as input
  pla1&2 as well : Gain  Gain=[0 0 0 0 0 0 0 0 1 1]  SaturateOnIntegerOverflow=on  OutDataTypeStr=Inherit: Same as input  ParamDataTypeStr=Inherit: Same as input
  controller output : Outport
  wires:
  inputs/1 -> pla1&2 as well/1
  state/1 -> VTAS sel/1
  VTAS sel/1 -> Sum/2  "VTAS"
  VTAS ref (trim value)/1 -> Sum/1
  Sum/1 -> Gain/1
  pla1&2/1 -> controller output is later added to pilot input!/1
  Gain/1 -> Saturation/1
  controller output is later added to pilot input!/1 -> controller output/1
  Saturation/1 -> pla1&2/1
  pla1&2 as well/1 -> controller output is later added to pilot input!/2

== system Citation_FlightGear_v2/FlightGear Visualisation/Subsystem/phidot thetadot psidot ==
  phi theta psi : Inport
  pqr : Inport  Port=2
  Concatenate1 : Concatenate  NumInputs=3
  Concatenate2 : Concatenate  NumInputs=3
  SinCos : aerolibobsolete/SinCos
  phidot : Fcn  Expr=u[1]+(u[2]*u[4]+u[3]*u[7])*(u[5]/u[8])
  psidot : Fcn  Expr=(u[2]*u[4]+u[3]*u[7])/u[8]
  thetadot : Fcn  Expr=u[2]*u[7]-u[3]*u[4]
  ptp_earth : Outport  VectorParamsAs1DForOutWhenUnconnected=off
  ptp_dot : Outport  Port=2  VectorParamsAs1DForOutWhenUnconnected=off
  wires:
  Concatenate1/1 -> psidot/1, phidot/1, thetadot/1
  pqr/1 -> Concatenate1/1
  phi theta psi/1 -> SinCos/1, ptp_earth/1
  psidot/1 -> Concatenate2/3
  thetadot/1 -> Concatenate2/2
  phidot/1 -> Concatenate2/1
  Concatenate2/1 -> ptp_dot/1
  SinCos/1 -> Concatenate1/2
  SinCos/2 -> Concatenate1/3

== system Citation_FlightGear_v2/Pilot/Virtual Joystick (if you don't have a real one!)/Virtual Joystick ==
  Add : Sum  Inputs=+++
  Throttle setting : Subsystem  Tag=STV Subsys  LoadFcn=sigbuilder_block('load');  StartFcn=sigbuilder_block('start');  StopFcn=sigbuilder_block('stop');  ClipboardFcn=sigbuilder_block('clipboard');  mask(Sigbuilder block){tuvar=[0:10]}
      mask help: Simulink:masks:SigbuilderBlock_MD
      mask init:
      | if ~strcmp(get_param(bdroot(gcbh),'SimulationStatus'),'stopped') tuvar = sigbuilder_block('maskInit'); end
      settings: CopyFcn=sigbuilder_block('copy');  DeleteFcn=sigbuilder_block('delete');  ModelCloseFcn=sigbuilder_block('modelClose');  PreSaveFcn=sigbuilder_block('preSave');  PauseFcn=sigbuilder_block('pause');  ContinueFcn=sigbuilder_block('continue');  NameChangeFcn=sigbuilder_block('namechange');  OpenFcn=sigbuilder_block('open',[241.5 168 795.75 479.25 ]);  CloseFcn=sigbuilder_block('close');
      mask Display: plot(0, 0, 100, 100,[2, 2, 32, 32, 2], [68, 8, 8, 68, 68],[32, 2], [38, 38], [32, 19, 2],[53, 60, 44], [32, 17, 17, 2],[16, 16, 31, 31]);txt = getActiveGroup(gcbh);text(2, 100, txt,'verticalAlignment', 'top');
  delta aileron : Subsystem  Tag=STV Subsys  LoadFcn=sigbuilder_block('load');  StartFcn=sigbuilder_block('start');  StopFcn=sigbuilder_block('stop');  ClipboardFcn=sigbuilder_block('clipboard');  mask(Sigbuilder block){tuvar=[0:10]}
      mask help: Simulink:masks:SigbuilderBlock_MD
      mask init:
      | if ~strcmp(get_param(bdroot(gcbh),'SimulationStatus'),'stopped') tuvar = sigbuilder_block('maskInit'); end
      settings: CopyFcn=sigbuilder_block('copy');  DeleteFcn=sigbuilder_block('delete');  ModelCloseFcn=sigbuilder_block('modelClose');  PreSaveFcn=sigbuilder_block('preSave');  PauseFcn=sigbuilder_block('pause');  ContinueFcn=sigbuilder_block('continue');  NameChangeFcn=sigbuilder_block('namechange');  OpenFcn=sigbuilder_block('open',[241.5 168 795.75 479.25 ]);  CloseFcn=sigbuilder_block('close');
      mask Display: plot(0, 0, 100, 100,[2, 2, 32, 32, 2], [68, 8, 8, 68, 68],[32, 2], [38, 38], [32, 19, 2],[53, 60, 44], [32, 17, 17, 2],[16, 16, 31, 31]);txt = getActiveGroup(gcbh);text(2, 100, txt,'verticalAlignment', 'top');
  delta elevator : Subsystem  Tag=STV Subsys  LoadFcn=sigbuilder_block('load');  StartFcn=sigbuilder_block('start');  StopFcn=sigbuilder_block('stop');  ClipboardFcn=sigbuilder_block('clipboard');  mask(Sigbuilder block){tuvar=[0:10]}
      mask help: Simulink:masks:SigbuilderBlock_MD
      mask init:
      | if ~strcmp(get_param(bdroot(gcbh),'SimulationStatus'),'stopped') tuvar = sigbuilder_block('maskInit'); end
      settings: CopyFcn=sigbuilder_block('copy');  DeleteFcn=sigbuilder_block('delete');  ModelCloseFcn=sigbuilder_block('modelClose');  PreSaveFcn=sigbuilder_block('preSave');  PauseFcn=sigbuilder_block('pause');  ContinueFcn=sigbuilder_block('continue');  NameChangeFcn=sigbuilder_block('namechange');  OpenFcn=sigbuilder_block('open',[241.5 168 795.75 479.25 ]);  CloseFcn=sigbuilder_block('close');
      mask Display: plot(0, 0, 100, 100,[2, 2, 32, 32, 2], [68, 8, 8, 68, 68],[32, 2], [38, 38], [32, 19, 2],[53, 60, 44], [32, 17, 17, 2],[16, 16, 31, 31]);txt = getActiveGroup(gcbh);text(2, 100, txt,'verticalAlignment', 'top');
  delta rudder : Subsystem  Tag=STV Subsys  LoadFcn=sigbuilder_block('load');  StartFcn=sigbuilder_block('start');  StopFcn=sigbuilder_block('stop');  ClipboardFcn=sigbuilder_block('clipboard');  mask(Sigbuilder block){tuvar=[0:10]}
      mask help: Simulink:masks:SigbuilderBlock_MD
      mask init:
      | if ~strcmp(get_param(bdroot(gcbh),'SimulationStatus'),'stopped') tuvar = sigbuilder_block('maskInit'); end
      settings: CopyFcn=sigbuilder_block('copy');  DeleteFcn=sigbuilder_block('delete');  ModelCloseFcn=sigbuilder_block('modelClose');  PreSaveFcn=sigbuilder_block('preSave');  PauseFcn=sigbuilder_block('pause');  ContinueFcn=sigbuilder_block('continue');  NameChangeFcn=sigbuilder_block('namechange');  OpenFcn=sigbuilder_block('open',[241.5 168 795.75 479.25 ]);  CloseFcn=sigbuilder_block('close');
      mask Display: plot(0, 0, 100, 100,[2, 2, 32, 32, 2], [68, 8, 8, 68, 68],[32, 2], [38, 38], [32, 19, 2],[53, 60, 44], [32, 17, 17, 2],[16, 16, 31, 31]);txt = getActiveGroup(gcbh);text(2, 100, txt,'verticalAlignment', 'top');
  Signal 1 : Outport
  Signal 2 : Outport  Port=2
  Signal 3 : Outport  Port=3
  Signal 4 : Outport  Port=4
  wires:
  delta elevator/1(Signal 1) -> Signal 1/1
  delta rudder/1(Signal 1) -> Signal 3/1
  Throttle setting/1(Signal 1) -> Signal 4/1
  delta aileron/1(Signal 1) -> Add/1
  Add/1 -> Signal 2/1
  delta aileron/2(Signal 2) -> Add/2
  delta aileron/3(Signal 3) -> Add/3

== system Citation_FlightGear_v2/Cessna Citation 500/Citation model DASMAT/AIRCRAFT MODEL/AFM ==
  x : Inport
  ua : Inport  Port=2
  massinit : Inport  Port=3
  yad1 : Inport  Port=4
  yad2 : Inport  Port=5
  gust : Inport  Port=6
  yatm : Inport  Port=7
  Aero axes-cg transformation : Subsystem
  Aeromod : Subsystem
  FMaerodims : Subsystem
  FMgustdims : Subsystem
  Gust axes-cg transformation : Subsystem
  FMa : Outport
  FMadot : Outport  Port=2
  FMbdot : Outport  Port=3
  FMag : Outport  Port=4
  wires:
  FMaerodims/3(FMbdot) -> FMbdot/1
  FMgustdims/1(FMag) -> FMag/1
  FMaerodims/2(FMadot) -> FMadot/1
  FMaerodims/1(FMa) -> FMa/1
  ua/1 -> Aeromod/2(ua)
  yad2/1 -> Aeromod/5(yad2)
  gust/1 -> Aeromod/6(gust)
  Aero axes-cg transformation/1(Ca) -> FMaerodims/1(Ca)
  Aero axes-cg transformation/2(Cadot) -> FMaerodims/2(Cadot)
  Aero axes-cg transformation/3(Cbdot) -> FMaerodims/3(Cbdot)
  Gust axes-cg transformation/1(Cag) -> FMgustdims/1(Cag)
  yad1/1 -> FMaerodims/5(yad1), FMgustdims/2(yad1), Aeromod/4(yad1)
  massinit/1 -> Aero axes-cg transformation/5(massinit), Gust axes-cg transformation/3(massinit), Aeromod/3(massinit)
  Aeromod/1(Ca) -> Aero axes-cg transformation/1(Ca model)
  Aeromod/2(Cadot) -> Aero axes-cg transformation/2(Cadot model)
  Aeromod/3(Cbdot) -> Aero axes-cg transformation/3(Cbdot model)
  Aeromod/4(Cag) -> Gust axes-cg transformation/1(Cag model)
  x/1 -> Aero axes-cg transformation/4("x "), Gust axes-cg transformation/2("x "), FMaerodims/4(x), Aeromod/1(x)
  yatm/1 -> Aeromod/7(yatm)

== system Citation_FlightGear_v2/Cessna Citation 500/Citation model DASMAT/AIRCRAFT MODEL/AIRDATA ==
  x : Inport
  terrain elevation : Inport  Port=2
  Demux : Demux  Outputs=[8 2 8]
      settings: DisplayOption=none
  Demux1 : Demux  Outputs=[5 1 2]
      settings: DisplayOption=none
  Mux : Mux  Inputs=[5 1 2]
  Sum : Sum  Inputs=-+|  SaturateOnIntegerOverflow=on
  airdata : S-Function  FunctionName=ac_atmos  SFunctionDeploymentMode=off  EnableBusSupport=off
  yatm : Outport
  yad1 : Outport  Port=2
  yad2 : Outport  Port=3
  wires:
  x/1 -> airdata/1
  airdata/1 -> Demux/1
  Demux/2 -> yad1/1
  Demux/3 -> yad2/1
  Demux/1 -> Demux1/1
  Mux/1 -> yatm/1
  Demux1/1 -> Mux/1
  Demux1/3 -> Mux/3
  Demux1/2 -> Sum/2
  Sum/1 -> Mux/2
  terrain elevation/1 -> Sum/1

== system Citation_FlightGear_v2/Cessna Citation 500/Citation model DASMAT/AIRCRAFT MODEL/EFM ==
  x : Inport
  ut : Inport  Port=2
  massinit : Inport  Port=3
  yatm : Inport  Port=4
  yad1 : Inport  Port=5
  yad2 : Inport  Port=6
  Engine axes-cg transformation : Subsystem
  Engmod : Subsystem
  FMt : Outport
  ypp : Outport  Port=2
  wires:
  massinit/1 -> Engine axes-cg transformation/3(massinit)
  Engine axes-cg transformation/1(FMt) -> FMt/1
  ut/1 -> Engmod/2(ut)
  yatm/1 -> Engmod/3(yatm)
  yad2/1 -> Engmod/5(yad2)
  x/1 -> Engine axes-cg transformation/2("x "), Engmod/1(x)
  yad1/1 -> Engmod/4(yad1)
  Engmod/1(FMt) -> Engine axes-cg transformation/1(FMt model)
  Engmod/2(ypp) -> ypp/1
